simulink model "c221007_FCEV_CDCS"  (R2022b)
settings: Solver=ode4  StartTime=1  StopTime=size(Driving_cycle_v_kmph,1)  FixedStep=Auto  RelTol=1e-3  EnableMultiTasking=on
values from neighbouring files (symbols this model uses):
  Bat_eff_chg_average = 0.969    [FCEV_original_data.mat]
  Bat_eff_dis_average = 0.9632    [FCEV_original_data.mat]
  Bat_end_of_life_percent = 20    [FCEV_original_data.mat]
  Bat_I_chg_max = -120    [FCEV_original_data.mat]
  Bat_I_dis_max = 200    [FCEV_original_data.mat]
  Bat_nom_Ic = 2.5    [FCEV_original_data.mat]
  Bat_nom_SOC = 0.35    [FCEV_original_data.mat]
  Bat_nom_temp_oC = 25    [FCEV_original_data.mat]
  Bat_num_pa = 9    [FCEV_original_data.mat]
  Bat_num_se = 97    [FCEV_original_data.mat]
  Bat_ori_C1_chg_F = [397.526659684 455.660832136 435.08783522 460.845064365 457.605812374 417.289828504 416.373906992 359.741413056 321.561704819 1109.14132554 1165.67733205 1135.97600211 ... (72 elements, 9x8)]    [FCEV_original_data.mat]
  Bat_ori_C1_dis_F = [187.121968588 287.083505726 346.448009002 395.529439835 387.517274826 389.973134196 432.856765051 486.92921923 512.158935268 425.990733989 614.68708868 771.472592368 ... (72 elements, 9x8)]    [FCEV_original_data.mat]
  Bat_ori_C2_chg_F = [8748.48589695 7773.35875681 9404.86567646 8934.73981058 8290.58671366 7592.78422269 7759.44623103 7396.59043829 6151.35152293 16187.7227039 11721.8480541 13157.8579836 ... (72 elements, 9x8)]    [FCEV_original_data.mat]
  Bat_ori_C2_dis_F = [2939.81325553 4590.73311898 5504.93546413 5887.5077374 6534.37836712 7765.46899768 10584.7751706 10372.0508438 9238.72693885 5207.86390693 7911.43744944 8879.62137571 ... (72 elements, 9x8)]    [FCEV_original_data.mat]
  Bat_ori_cap_max_Ah = 20.7    [Config_c221218.m]    (also in Config_c230117.m; Config_c230321.m; FCEV_original_data.mat)
  Bat_ori_dUdt4 = [-0.303773584906 -0.249056603774 -0.115094339623 -0.0396226415094 0.0396226415094 0.0641509433962 0.107547169811 0.111320754717 0.0415094339623 0.0547169811321 0.130188679245]    [FCEV_original_data.mat]
  Bat_ori_R0_chg_O = [0.0771669453735 0.0731809311402 0.0726556782939 0.0729965156794 0.0731758310684 0.0742031005051 0.0721266921026 0.0714211058078 0.0714186176143 0.0374124505155 0.0354566732504 0.0345430657188 ... (72 elements, 9x8)]    [FCEV_original_data.mat]
  Bat_ori_R0_dis_O = [0.0819458671157 0.0812429476608 0.0803749674507 0.0805513601722 0.0838629023857 0.0850797840015 0.0829875518672 0.0826388888889 0.0812514106148 0.0428124986417 0.0424658903711 0.0428572670451 ... (72 elements, 9x8)]    [FCEV_original_data.mat]
  Bat_ori_R1_chg_O = [0.114339870884 0.105392753268 0.104421193553 0.109821896183 0.114868279838 0.123333154908 0.129174812826 0.149917249373 0.174896487845 0.0420560161846 0.0390948352938 0.0370122837364 ... (72 elements, 9x8)]    [FCEV_original_data.mat]
  Bat_ori_R1_dis_O = [0.304806399643 0.213604089624 0.171463520004 0.151183840498 0.140630862434 0.128795299077 0.116857791733 0.112567113582 0.106368362501 0.0943235089866 0.0730697254134 0.0611414736086 ... (72 elements, 9x8)]    [FCEV_original_data.mat]
  Bat_ori_R2_chg_O = [0.134518959939 0.17565045702 0.161100627268 0.189032232545 0.205639040497 0.226170473035 0.223651875822 0.181765694192 0.212966950836 0.073628872144 0.0788540822416 0.0792414571734 ... (72 elements, 9x8)]    [FCEV_original_data.mat]
  Bat_ori_R2_dis_O = [0.354968099904 0.285293035102 0.286338708953 0.298763853987 0.248762838155 0.178586175471 0.129047399775 0.188406991173 0.174494800676 0.131839238891 0.123225430215 0.132069033134 ... (72 elements, 9x8)]    [FCEV_original_data.mat]
  Bat_ori_SOC2 = [0 0.001 0.002 0.003 0.004 0.005 0.006 0.007 0.008 0.009 0.01 0.011 ... (1001 elements, 1x1001)]    [FCEV_original_data.mat]
  Bat_ori_SOC4 = [-0.00598301069999 0.0920117618231 0.190864167279 0.289083557951 0.387343788287 0.485011843502 0.5850485992 0.678163031937 0.774810095565 0.876684636119 0.972739524626]    [FCEV_original_data.mat]
  Bat_ori_Uoc_chg_V = [2.4478 2.54923264342 2.6007 2.6383 2.66953057366 2.69636321708 2.7197 2.74042850391 2.75906114733 2.77619379074 2.792 2.80675907757 ... (1001 elements, 1x1001)]    [FCEV_original_data.mat]
  Bat_ori_Uoc_dis_V = [1.9998 2.03916768329 2.24724374236 2.39700902919 2.48767431602 2.5476 2.5882 2.6202 2.64771773167 2.6719 2.6933 2.71251566192 ... (1001 elements, 1x1001)]    [FCEV_original_data.mat]
  Bat_ori_Uoc_V = [2.2238 2.29420016335 2.42397187118 2.5176545146 2.57860244484 2.62198160854 2.65395 2.68031425195 2.7033894395 2.72404689537 2.74265 2.75963736975 ... (1001 elements, 1x1001)]    [FCEV_original_data.mat]
  Bat_single_capacity_nom_Ah = 2.3    [FCEV_original_data.mat]
  Bat_SOC_cs_max = 0.4    [FCEV_original_data.mat]
  Bat_SOC_cs_min = 0.2    [FCEV_original_data.mat]
  Bat_SOC_ini = 0.3    [Config_c22100601.m]    (also in Config_c22100701.m; FCEV_original_data.mat = 0.45)
  Bat_SOC_max = 0.9    [FCEV_original_data.mat]
  Bat_SOC_min = 0.3    [FCEV_original_data.mat]
  Bat_temp_amb_oC = 25    [FCEV_original_data.mat]
  Bat_temp_cool_oC = 25    [FCEV_original_data.mat]
  Bat_U_avg_V = Bat_num_se*mean(Bat_ori_Uoc_V)    [Config_c22100601.m]    (also in Config_c22100701.m)
  DCAC_eff = 0.95    [FCEV_original_data.mat]
  DCDC_ori_eff = [0.95 0.96 0.97 0.976 0.98 0.978 0.973 0.962]    [FCEV_original_data.mat]
  DCDC_ori_power_kW = [0 10 20 30 40 50 60 70]    [FCEV_original_data.mat]
  FC_fuel_mass_ini_kg = 10    [FCEV_original_data.mat]
  FC_ori_eff = [0.1 0.33 0.492 0.533 0.559 0.596 0.591 0.562 0.508]    [FCEV_original_data.mat]
  FC_ori_fuel_rate_gps = [0 0.0505050505051 0.0846883468835 0.117260787992 0.149075730471 0.279642058166 0.423011844332 0.593119810202 0.820209973753]    [FCEV_original_data.mat]
  FC_ori_power_kW = [0 2 5 7.5 10 20 30 40 50]    [FCEV_original_data.mat]
  FC_power_max_kW = 50    [FCEV_original_data.mat]
  FC_power_min_kW = 0    [FCEV_original_data.mat]
  MC_eff_brk_average = 0.810578512397    [FCEV_original_data.mat]
  MC_eff_dri_average = 0.810578512397    [FCEV_original_data.mat]
  MC_inertia = 0.06    [FCEV_original_data.mat]
  MC_ori_eff = [0.7 0.78 0.85 0.86 0.81 0.82 0.79 0.78 0.78 0.78 0.78 0.7 ... (231 elements, 11x21)]    [FCEV_original_data.mat]
  MC_ori_power_brk_req_kW = [0 -28.3912930389 -56.7825860779 -85.1738791168 -113.565172156 -141.956465195 -170.347758234 -198.739051273 -227.130344311 -255.52163735 -283.912930389 0 ... (121 elements, 11x11)]    [FCEV_original_data.mat]
  MC_ori_power_dri_req_kW = [0 0 0 0 0 0 0 0 0 0 0 0 ... (121 elements, 11x11)]    [FCEV_original_data.mat]
  MC_ori_spd_rpm = [0 1000 2000 3000 4000 5000 6000 7000 8000 9000 10000]    [FCEV_original_data.mat]
  MC_ori_trq_brk_max_Nm = [-271.1368 -271.1368 -271.1368 -237.5159 -178.1369 -142.4824 -118.7579 -101.8119 -89.0685 -79.172 -71.1734]    [FCEV_original_data.mat]
  MC_ori_trq_brk_Nm = [-271.136848522 -244.02316367 -216.909478817 -189.795793965 -162.682109113 -135.568424261 -108.454739409 -81.3410545565 -54.2273697044 -27.1136848522 0]    [FCEV_original_data.mat]
  MC_ori_trq_dri_max_Nm = [271.1368 271.1368 271.1368 237.5159 178.1369 142.4824 118.7579 101.8119 89.0685 79.172 71.1734]    [FCEV_original_data.mat]
  MC_ori_trq_dri_Nm = [0 27.1136848522 54.2273697044 81.3410545565 108.454739409 135.568424261 162.682109113 189.795793965 216.909478817 244.02316367 271.136848522]    [FCEV_original_data.mat]
  MC_ori_trq_Nm = [-271.136848522 -244.02316367 -216.909478817 -189.795793965 -162.682109113 -135.568424261 -108.454739409 -81.3410545565 -54.2273697044 -27.1136848522 0 27.1136848522 ... (21 elements, 1x21)]    [FCEV_original_data.mat]
  MC_power_max_kW = 75    [FCEV_original_data.mat]
  MC_spd_max_rpm = 10000    [FCEV_original_data.mat]
  MC_spd_min_rpm = 0    [FCEV_original_data.mat]
  MC_spd_scale = 1    [FCEV_original_data.mat]
  MC_trq_scale = 1    [FCEV_original_data.mat]
  MC_U_min_V = 120    [FCEV_original_data.mat]
  Road_u = 0.75    [FCEV_original_data.mat]
  S_r = floor(max(Sr_SOC_process(:,1))):-1:0    [Config_c22100601.m]    (also in Config_c22100701.m)
  Time_sample = 60    [Driving_cycle_recognition_data.mat]
  Trip_distance_total_km = sum(Driving_cycle_v_kmph(:,2)/3.6)/1000    [Config_c22100601.m]    (also in Config_c22100701.m)
  usd2rmb = 7.116    [Config_c22100601.m]    (also in Config_c22100701.m; Config_c221106.m = 6; Config_c221112.m = 6; Config_c221127.m = 6)
  Veh_air_density_kgpm2 = 1.2    [FCEV_original_data.mat]
  Veh_brk_front = [1 0.6 0.608 0.61 0.618 0.624 0.636 0.645 0.655]    [FCEV_original_data.mat]
  Veh_brk_z = [0.1 0.2 0.3 0.4 0.5 0.6 0.7 0.8 0.9]    [FCEV_original_data.mat]
  Veh_brk_z_max = 0.7    [FCEV_original_data.mat]
  Veh_brk_z_min = 0.1    [FCEV_original_data.mat]
  Veh_coeff_drag = 0.312    [FCEV_original_data.mat]
  Veh_coeff_roll = 0.00863    [FCEV_original_data.mat]
  Veh_final_drive_inertia = 0.1105    [FCEV_original_data.mat]
  Veh_final_drive_ratio = 3.47    [FCEV_original_data.mat]
  Veh_frontal_area_m2 = 2.06    [FCEV_original_data.mat]
  Veh_gravity_acc_ms2 = 9.81    [FCEV_original_data.mat]
  Veh_mass_cargo_kg = 113    [FCEV_original_data.mat]
  Veh_mass_curb_kg = 1157    [FCEV_original_data.mat]
  Veh_mech_eff = 0.9    [FCEV_original_data.mat]
  Veh_rotary_mass_conversion_factor = 1.05    [FCEV_original_data.mat]
  Veh_size_cg_height_m = 0.53    [FCEV_original_data.mat]
  Veh_wheel_inertia = 3.1039    [FCEV_original_data.mat]
  Veh_wheel_radius_m = 0.313    [FCEV_original_data.mat]
  Veh_wt_frac_front = 0.5    [FCEV_original_data.mat]
undefined symbols (not defined in the file or in its folder): alpha, Bat_ori_temp, Sr_e
libraries: neural x10
(part 4 of 5)

== system c221007_FCEV_CDCS/电池模型/Electrical Model/Max power in W (Battery pack level)/Max power in W (Battery pack level)1 ==
  SOC : Inport
  1-D Lookup Table : Lookup_n-D  NumberOfTableDimensions=1  BreakpointsForDimension1=Bat_ori_SOC2  Table=Bat_ori_Uoc_V  RndMeth=Simplest
  1-D Lookup Table1 : Lookup_n-D  NumberOfTableDimensions=1  BreakpointsForDimension1=Bat_ori_SOC2  Table=Bat_ori_Uoc_V  RndMeth=Simplest
  Constant : Constant  Value=MC_U_min_V
  Constant1 : Constant  Value=0.001
  Constant2 : Constant  Value=0
  Constant3 : Constant  Value=Bat_SOC_min
  Constant4 : Constant  Value=Bat_SOC_max
  Gain : Gain  Gain=0.5  SaturateOnIntegerOverflow=on  OutDataTypeStr=Inherit: Same as input  ParamDataTypeStr=Inherit: Same as input
  MinMax1 : MinMax  Function=max  Inputs=3  InputSameDT=on  SaturateOnIntegerOverflow=on
  Mux : Mux  Inputs=3
  Mux3 : Mux  Inputs=3
  Mux5 : Mux  Inputs=3
  Product3 : Product  InputSameDT=on  RndMeth=Zero  SaturateOnIntegerOverflow=on  OutDataTypeStr=Inherit: Same as first input
  R0,cell->R0,bat : Gain  Gain=Bat_num_se/Bat_num_pa  SaturateOnIntegerOverflow=on  OutDataTypeStr=Inherit: Same as input  ParamDataTypeStr=Inherit: Same as input
  R0,cell->R0,bat1 : Gain  Gain=Bat_num_se/Bat_num_pa  SaturateOnIntegerOverflow=on  OutDataTypeStr=Inherit: Same as input  ParamDataTypeStr=Inherit: Same as input
  Relational Operator : RelationalOperator  Operator=>
  Switch : Switch  Threshold=eps
  Uoc,cell->Uoc,bat : Gain  Gain=Bat_num_se  SaturateOnIntegerOverflow=on  OutDataTypeStr=Inherit: Same as input  ParamDataTypeStr=Inherit: Same as input
  Uoc,cell->Uoc,bat1 : Gain  Gain=Bat_num_se  SaturateOnIntegerOverflow=on  OutDataTypeStr=Inherit: Same as input  ParamDataTypeStr=Inherit: Same as input
  Voc-I*R : Fcn  Expr=u[2]-u[1]*u[3]
  iabs min=(Voc-Vmax)/R : Fcn  Expr=(u(1)-u(2))/u(3)
  max power corresponding to minimum voltage : Fcn  Expr=(u[1]-u[2])*u[2]/u[3]
  max ess discharge pwr : Outport  InitialOutput=0
  max ess charge pwr : Outport  Port=2  InitialOutput=0
  wires:
  Voc-I*R/1 -> Product3/2
  iabs min=(Voc-Vmax)/R/1 -> Product3/1, Mux3/1
  Mux3/1 -> Voc-I*R/1
  Mux5/1 -> iabs min=(Voc-Vmax)/R/1
  Uoc,cell->Uoc,bat1/1 -> Mux5/2
  Switch/1 -> max ess discharge pwr/1
  SOC/1 -> Relational Operator/1
  Constant2/1 -> Switch/3
  max power corresponding to minimum voltage/1 -> Switch/1
  [Bat_Uoc_V] -> Mux3/2, Mux5/1, Gain/1, Mux/1
  MinMax1/1 -> Mux/2
  Gain/1 -> MinMax1/1
  Mux/1 -> max power corresponding to minimum voltage/1
  Constant/1 -> MinMax1/2
  Constant1/1 -> Relational Operator/2
  Uoc,cell->Uoc,bat/1 -> MinMax1/3
  Relational Operator/1 -> Switch/2
  [Bat_R0_dis_O] -> R0,cell->R0,bat/1
  R0,cell->R0,bat/1 -> Mux/3
  [Bat_R0_chg_O] -> R0,cell->R0,bat1/1
  R0,cell->R0,bat1/1 -> Mux5/3, Mux3/3
  Constant3/1 -> 1-D Lookup Table/1
  1-D Lookup Table/1 -> Uoc,cell->Uoc,bat/1
  Constant4/1 -> 1-D Lookup Table1/1
  1-D Lookup Table1/1 -> Uoc,cell->Uoc,bat1/1
  Product3/1 -> max ess charge pwr/1

== system c221007_FCEV_CDCS/电池模型/Electrical Model/Parameter Lookup2/Lookup C1 ==
  SOC : Inport
  T : Inport  Port=2
  P : Inport  Port=3
  Lookup Table (2-D) C1_c : Lookup2D  RowIndex=Bat_ori_SOC_chg  ColumnIndex=Bat_ori_temp_oC  Table=Bat_ori_C1_chg_F  SaturateOnIntegerOverflow=off  InputSameDT=off
  Lookup Table (2-D) C1_d : Lookup2D  RowIndex=Bat_ori_SOC_dis  ColumnIndex=Bat_ori_temp_oC  Table=Bat_ori_C1_dis_F  SaturateOnIntegerOverflow=off  InputSameDT=off
  Switch : Switch  SaturateOnIntegerOverflow=off  InputSameDT=off
  C1 : Outport
  wires:
  T/1 -> Lookup Table (2-D) C1_c/2, Lookup Table (2-D) C1_d/2
  SOC/1 -> Lookup Table (2-D) C1_c/1, Lookup Table (2-D) C1_d/1
  Lookup Table (2-D) C1_c/1 -> Switch/3
  Lookup Table (2-D) C1_d/1 -> Switch/1
  Switch/1 -> C1/1
  P/1 -> Switch/2

== system c221007_FCEV_CDCS/电池模型/Electrical Model/Parameter Lookup2/Lookup C2 ==
  SOC : Inport
  T : Inport  Port=2
  P : Inport  Port=3
  Lookup Table (2-D) C2_c : Lookup2D  RowIndex=Bat_ori_SOC_chg  ColumnIndex=Bat_ori_temp_oC  Table=Bat_ori_C2_chg_F  SaturateOnIntegerOverflow=off  InputSameDT=off
  Lookup Table (2-D) C2_d : Lookup2D  RowIndex=Bat_ori_SOC_dis  ColumnIndex=Bat_ori_temp_oC  Table=Bat_ori_C2_dis_F  SaturateOnIntegerOverflow=off  InputSameDT=off
  Switch : Switch  SaturateOnIntegerOverflow=off  InputSameDT=off
  C2 : Outport
  wires:
  T/1 -> Lookup Table (2-D) C2_c/2, Lookup Table (2-D) C2_d/2
  SOC/1 -> Lookup Table (2-D) C2_c/1, Lookup Table (2-D) C2_d/1
  Lookup Table (2-D) C2_c/1 -> Switch/3
  Lookup Table (2-D) C2_d/1 -> Switch/1
  Switch/1 -> C2/1
  P/1 -> Switch/2

== system c221007_FCEV_CDCS/电池模型/Electrical Model/Parameter Lookup2/Lookup R1 ==
  SOC : Inport
  T : Inport  Port=2
  P : Inport  Port=3
  Lookup Table (2-D) R1_c : Lookup2D  RowIndex=Bat_ori_SOC_chg  ColumnIndex=Bat_ori_temp_oC  Table=Bat_ori_R1_chg_O  SaturateOnIntegerOverflow=off  InputSameDT=off
  Lookup Table (2-D) R1_d : Lookup2D  RowIndex=Bat_ori_SOC_dis  ColumnIndex=Bat_ori_temp_oC  Table=Bat_ori_R1_dis_O  SaturateOnIntegerOverflow=off  InputSameDT=off
  Switch : Switch  SaturateOnIntegerOverflow=off  InputSameDT=off
  R1 : Outport
  wires:
  T/1 -> Lookup Table (2-D) R1_d/2, Lookup Table (2-D) R1_c/2
  SOC/1 -> Lookup Table (2-D) R1_d/1, Lookup Table (2-D) R1_c/1
  Lookup Table (2-D) R1_c/1 -> Switch/3
  Lookup Table (2-D) R1_d/1 -> Switch/1
  P/1 -> Switch/2
  Switch/1 -> R1/1

== system c221007_FCEV_CDCS/电池模型/Electrical Model/Parameter Lookup2/Lookup R2 ==
  SOC1 : Inport
  T : Inport  Port=2
  P : Inport  Port=3
  Lookup Table (2-D) R2_c : Lookup2D  RowIndex=Bat_ori_SOC_chg  ColumnIndex=Bat_ori_temp_oC  Table=Bat_ori_R2_chg_O  SaturateOnIntegerOverflow=off  InputSameDT=off
  Lookup Table (2-D) R2_d : Lookup2D  RowIndex=Bat_ori_SOC_dis  ColumnIndex=Bat_ori_temp_oC  Table=Bat_ori_R2_dis_O  SaturateOnIntegerOverflow=off  InputSameDT=off
  Switch : Switch  SaturateOnIntegerOverflow=off  InputSameDT=off
  R2 : Outport
  wires:
  T/1 -> Lookup Table (2-D) R2_d/2, Lookup Table (2-D) R2_c/2
  SOC1/1 -> Lookup Table (2-D) R2_d/1, Lookup Table (2-D) R2_c/1
  Lookup Table (2-D) R2_c/1 -> Switch/3
  Lookup Table (2-D) R2_d/1 -> Switch/1
  P/1 -> Switch/2
  Switch/1 -> R2/1

== system c221007_FCEV_CDCS/电池模型/Electrical Model/Parameter Lookup2/Lookup Rs ==
  SOC : Inport
  T : Inport  Port=2
  Lookup Table (2-D) R0_c : Lookup2D  RowIndex=Bat_ori_SOC_chg  ColumnIndex=Bat_ori_temp_oC  Table=Bat_ori_R0_chg_O  SaturateOnIntegerOverflow=off  InputSameDT=off
  Lookup Table (2-D) R0_d : Lookup2D  RowIndex=Bat_ori_SOC_dis  ColumnIndex=Bat_ori_temp_oC  Table=Bat_ori_R0_dis_O  SaturateOnIntegerOverflow=off  InputSameDT=off
  Mux : Mux  Inputs=2
  R0 : Outport
  tag scope: Bat_R0_chg_O=global, Bat_R0_dis_O=global
  wires:
  Lookup Table (2-D) R0_d/1 -> Mux/1, [Bat_R0_dis_O]
  Lookup Table (2-D) R0_c/1 -> Mux/2, [Bat_R0_chg_O]
  SOC/1 -> Lookup Table (2-D) R0_c/1, Lookup Table (2-D) R0_d/1
  T/1 -> Lookup Table (2-D) R0_c/2, Lookup Table (2-D) R0_d/2
  Mux/1 -> R0/1

== system c221007_FCEV_CDCS/电池模型/Electrical Model/Parameter Lookup2/Lookup Uoc ==
  SOC : Inport
  P : Inport  Port=2
  Switch : Switch  SaturateOnIntegerOverflow=off  InputSameDT=off
  VOC-chg : Lookup_n-D  NumberOfTableDimensions=1  BreakpointsForDimension1=Bat_ori_SOC2  BreakpointsForDimension2=Bat_ori_temp  Table=Bat_ori_Uoc_chg_V  InternalRulePriority=Speed  RndMeth=Simplest
  VOC-dischg : Lookup_n-D  NumberOfTableDimensions=1  BreakpointsForDimension1=Bat_ori_SOC2  BreakpointsForDimension2=Bat_ori_temp  Table=Bat_ori_Uoc_dis_V  InternalRulePriority=Speed  RndMeth=Simplest
  Uoc : Outport
  wires:
  SOC/1 -> VOC-chg/1, VOC-dischg/1
  VOC-chg/1 -> Switch/3
  VOC-dischg/1 -> Switch/1
  Switch/1 -> Uoc/1
  P/1 -> Switch/2

== system c221007_FCEV_CDCS/电池模型/Electrical Model/SOC Calculation/CD//CS mode judgement ==
  note: 当前SOC
  SOC : Inport
  Constant2 : Constant  Value=Bat_SOC_min
  Logical Operator1 : Logic  Operator=NOT  AllPortsSameDT=off  OutDataTypeStr=boolean
  Relational Operator : RelationalOperator  OutDataTypeStr=boolean  InputSameDT=off
  Scope1 : Scope
  To Workspace2 : ToWorkspace  VariableName=Bat_charge_sustaining_on  SampleTime=-1
  tag scope: Bat_charge_sustaining_on=global
  wires:
  SOC/1 -> Relational Operator/1
  Constant2/1 -> Relational Operator/2
  Logical Operator1/1 -> Scope1/1, To Workspace2/1, [Bat_charge_sustaining_on]
  Relational Operator/1 -> Logical Operator1/1

== system c221007_FCEV_CDCS/电池模型/Subsystem/Capacity Degradation Model (Cell)1/计算实际寿命 ==
  note: 参考文献：A control-oriented cycle-life model for hybrid electric vehicle lithiumion batteries
  note: Beta
  note: Alpha
  温度 : Inport
  倍率 : Inport  Port=2
  SOC : Inport  Port=3
  -31700+163.3*Ic : Sum  InputSameDT=on  SaturateOnIntegerOverflow=on  OutDataTypeStr=Inherit: Same as first input
  Alpha*SOC+Beta1 : Sum  InputSameDT=on  SaturateOnIntegerOverflow=on  OutDataTypeStr=Inherit: Same as first input
  Alpha3 : Constant  Value=2896.6
  Alpha4 : Constant  Value=2649.5
  Beta3 : Constant  Value=7411.2
  Beta4 : Constant  Value=6022.2
  Constant : Constant  Value=-31500
  Constant1 : Constant  Value=152.5
  Constant2 : Constant  Value=273.15
  Fcn2 : Fcn  Expr=u^(1/0.57)
  Math Function : Math  Operator=reciprocal  SignedPower=on
  Math Function1 : Math  Operator=reciprocal  SignedPower=on
  Math Function2 : Math  SignedPower=on
  R : Constant  Value=8.314
  R*T : Product  InputSameDT=on  RndMeth=Zero  SaturateOnIntegerOverflow=on  OutDataTypeStr=Inherit: Same as first input
  Switch3 : Switch  Criteria=u2 > Threshold  Threshold=0.45
  Switch4 : Switch  Criteria=u2 > Threshold  Threshold=0.45
  severity factor function : Product  InputSameDT=on  RndMeth=Zero  SaturateOnIntegerOverflow=on  OutDataTypeStr=Inherit: Same as first input
  x : Product  InputSameDT=on  RndMeth=Zero  SaturateOnIntegerOverflow=on  OutDataTypeStr=Inherit: Same as first input
  x1 : Product  InputSameDT=on  RndMeth=Zero  SaturateOnIntegerOverflow=on  OutDataTypeStr=Inherit: Same as first input
  x2 : Product  InputSameDT=on  RndMeth=Zero  SaturateOnIntegerOverflow=on  OutDataTypeStr=Inherit: Same as first input
  ×1 : Product  InputSameDT=on  RndMeth=Zero  SaturateOnIntegerOverflow=on  OutDataTypeStr=Inherit: Same as first input
  ℃->开氏温度(绝对温度) : Sum  InputSameDT=on  SaturateOnIntegerOverflow=on  OutDataTypeStr=Inherit: Same as first input
  电池标准状态寿命 : ToWorkspace  VariableName=Bat_life_nom  SampleTime=-1
  电池终止寿命(%) : Constant  Value=Bat_end_of_life_percent
  Bat_life_nom : Outport
  wires:
  R/1 -> R*T/1
  ℃->开氏温度(绝对温度)/1 -> R*T/2
  Constant/1 -> -31700+163.3*Ic/1
  x/1 -> -31700+163.3*Ic/2
  Constant1/1 -> x/1
  -31700+163.3*Ic/1 -> x1/1
  R*T/1 -> Math Function/1
  Math Function/1 -> x1/2
  x1/1 -> Math Function2/1
  温度/1 -> ℃->开氏温度(绝对温度)/1
  Constant2/1 -> ℃->开氏温度(绝对温度)/2
  倍率/1 -> x/2
  Math Function2/1 -> severity factor function/1
  Alpha*SOC+Beta1/1 -> severity factor function/2
  severity factor function/1 -> Math Function1/1
  电池终止寿命(%)/1 -> x2/1
  Math Function1/1 -> x2/2
  x2/1 -> Fcn2/1
  Fcn2/1 -> Bat_life_nom/1, 电池标准状态寿命/1
  SOC/1 -> Switch4/2, ×1/1, Switch3/2
  Alpha4/1 -> Switch3/1
  Alpha3/1 -> Switch3/3
  Beta4/1 -> Switch4/1
  Beta3/1 -> Switch4/3
  Switch3/1 -> ×1/2
  Switch4/1 -> Alpha*SOC+Beta1/2
  ×1/1 -> Alpha*SOC+Beta1/1

== system c221007_FCEV_CDCS/电池模型/Subsystem/Capacity Degradation Model (Cell)1/计算电池寿命(标准条件下) ==
  note: 参考文献：A control-oriented cycle-life model for hybrid electric vehicle lithiumion batteries
  note: Beta
  note: Alpha
  标准温度 : Inport
  标准倍率 : Inport  Port=2
  标准SOC : Inport  Port=3
  -31500+152.5*Ic : Sum  InputSameDT=on  SaturateOnIntegerOverflow=on  OutDataTypeStr=Inherit: Same as first input
  Alpha*SOC+Beta : Sum  InputSameDT=on  SaturateOnIntegerOverflow=on  OutDataTypeStr=Inherit: Same as first input
  Alpha3 : Constant  Value=2896.6
  Alpha4 : Constant  Value=2649.5
  Beta3 : Constant  Value=7411.2
  Beta4 : Constant  Value=6022.2
  Constant : Constant  Value=-31500
  Constant1 : Constant  Value=152.5
  Constant2 : Constant  Value=273.15
  Fcn2 : Fcn  Expr=u^(1/0.57)
  Math Function : Math  Operator=reciprocal  SignedPower=on
  Math Function1 : Math  Operator=reciprocal  SignedPower=on
  Math Function2 : Math  SignedPower=on
  R : Constant  Value=8.314
  R*T : Product  InputSameDT=on  RndMeth=Zero  SaturateOnIntegerOverflow=on  OutDataTypeStr=Inherit: Same as first input
  Switch3 : Switch  Criteria=u2 > Threshold  Threshold=0.45
  Switch4 : Switch  Criteria=u2 > Threshold  Threshold=0.45
  severity factor function : Product  InputSameDT=on  RndMeth=Zero  SaturateOnIntegerOverflow=on  OutDataTypeStr=Inherit: Same as first input
  x : Product  InputSameDT=on  RndMeth=Zero  SaturateOnIntegerOverflow=on  OutDataTypeStr=Inherit: Same as first input
  x1 : Product  InputSameDT=on  RndMeth=Zero  SaturateOnIntegerOverflow=on  OutDataTypeStr=Inherit: Same as first input
  x2 : Product  InputSameDT=on  RndMeth=Zero  SaturateOnIntegerOverflow=on  OutDataTypeStr=Inherit: Same as first input
  ×1 : Product  InputSameDT=on  RndMeth=Zero  SaturateOnIntegerOverflow=on  OutDataTypeStr=Inherit: Same as first input
  ℃->开氏温度(绝对温度) : Sum  InputSameDT=on  SaturateOnIntegerOverflow=on  OutDataTypeStr=Inherit: Same as first input
  电池实际状态寿命 : ToWorkspace  VariableName=Bat_life_act  SampleTime=-1
  电池终止寿命(%) : Constant  Value=Bat_end_of_life_percent
  Bat_life_act : Outport
  wires:
  R/1 -> R*T/1
  ℃->开氏温度(绝对温度)/1 -> R*T/2
  Constant/1 -> -31500+152.5*Ic/1
  x/1 -> -31500+152.5*Ic/2
  Constant1/1 -> x/1
  -31500+152.5*Ic/1 -> x1/1
  R*T/1 -> Math Function/1
  Math Function/1 -> x1/2
  x1/1 -> Math Function2/1
  标准温度/1 -> ℃->开氏温度(绝对温度)/1
  Constant2/1 -> ℃->开氏温度(绝对温度)/2
  标准倍率/1 -> x/2
  Math Function2/1 -> severity factor function/1
  Alpha*SOC+Beta/1 -> severity factor function/2
  severity factor function/1 -> Math Function1/1
  电池终止寿命(%)/1 -> x2/1
  Math Function1/1 -> x2/2
  x2/1 -> Fcn2/1
  Fcn2/1 -> Bat_life_act/1, 电池实际状态寿命/1
  标准SOC/1 -> Switch4/2, ×1/1, Switch3/2
  Alpha4/1 -> Switch3/1
  Alpha3/1 -> Switch3/3
  Beta4/1 -> Switch4/1
  Beta3/1 -> Switch4/3
  Switch3/1 -> ×1/2
  Switch4/1 -> Alpha*SOC+Beta/2
  ×1/1 -> Alpha*SOC+Beta/1

== system c221007_FCEV_CDCS/电池模型/Subsystem/Electrical Model1/Current calculation ==
  note: #:电池单体水平
  note: R0chg
  note: R0dis
  Voc : Inport
  Rint : Inport  Port=2
  limited output power (W) : Inport  Port=3
  Constant : Constant  Value=Bat_I_chg_max
  Constant1 : Constant  Value=Bat_I_dis_max
  Constant2 : Constant  Value=0
  Demux : Demux  Outputs=2
  Ibty=(Voc-(Voc^2-4RPbty)^.5) ----------------------------- (2*R) : Fcn  Expr=(u[2]-(u[2]^2-4*u[1]*u[3])^.5)/(2*u[3])
  Ibty=(Voc-(Voc^2-4RPbty)^.5) ----------------------------- (2*R)1 : Fcn  Expr=(u[2]-(u[2]^2-4*u[1]*u[3])^.5)/(2*u[3])
  MinMax : MinMax  Inputs=2
  MinMax1 : MinMax  Function=max  Inputs=2
  Mux : Mux  Inputs=2
  Mux1 : Mux  Inputs=3
  Mux2 : Mux  Inputs=3
  Pbat->Pcell : Gain  Gain=1/(Bat_num_pa*Bat_num_se)  SaturateOnIntegerOverflow=on  OutDataTypeStr=Inherit: Same as input  ParamDataTypeStr=Inherit: Same as input
  Scope : Scope
  Scope1 : Scope
  Switch : Switch  Criteria=u2 > Threshold
  Switch1 : Switch  Criteria=u2 > Threshold  SaturateOnIntegerOverflow=off  InputSameDT=off
  Switch2 : Switch  Criteria=u2 > Threshold
  I_dis (A) I_chg (A) Cell : Outport  InitialOutput=0
  I (A) Cell : Outport  Port=2  InitialOutput=0
  wires:
  Rint/1 -> Demux/1
  limited output power (W)/1 -> Pbat->Pcell/1
  Pbat->Pcell/1 -> Switch/1, Switch/2, Switch2/3, Switch2/2, Switch1/2
  Mux1/1 -> Ibty=(Voc-(Voc^2-4RPbty)^.5) ----------------------------- (2*R)/1
  Demux/1 -> Mux1/3
  Voc/1 -> Mux1/2, Mux2/2
  Demux/2 -> Mux2/3
  Mux2/1 -> Ibty=(Voc-(Voc^2-4RPbty)^.5) ----------------------------- (2*R)1/1
  Ibty=(Voc-(Voc^2-4RPbty)^.5) ----------------------------- (2*R)/1 -> MinMax/2
  Constant1/1 -> MinMax/1
  Ibty=(Voc-(Voc^2-4RPbty)^.5) ----------------------------- (2*R)1/1 -> MinMax1/1
  Constant/1 -> MinMax1/2
  MinMax/1 -> Switch1/1, Mux/1
  MinMax1/1 -> Mux/2, Switch1/3
  Mux/1 -> Scope/1, I_dis (A) I_chg (A) Cell/1
  Switch1/1 -> Scope1/1, I (A) Cell/1
  Switch/1 -> Mux1/1
  Switch2/1 -> Mux2/1
  Constant2/1 -> Switch/3, Switch2/1

== system c221007_FCEV_CDCS/电池模型/Subsystem/Electrical Model1/Entropic Heat ==
  note: 用于计算可逆热
  T : Inport
  SOC : Inport  Port=2
  Constant : Constant  Value=273
  Ent heat : Product  RndMeth=Zero
  Scope : Scope
  Sum2 : Sum  Inputs=|++
  dudT : Lookup  InputValues=Bat_ori_SOC4  Table=Bat_ori_dUdt4  SaturateOnIntegerOverflow=off
  mV->V : Gain  Gain=1/1000
  HG_ent : Outport
  wires:
  Sum2/1 -> Ent heat/2
  Constant/1 -> Sum2/2
  T/1 -> Sum2/1
  dudT/1 -> Ent heat/1
  Ent heat/1 -> mV->V/1
  SOC/1 -> dudT/1
  mV->V/1 -> Scope/1, HG_ent/1

== system c221007_FCEV_CDCS/电池模型/Subsystem/Electrical Model1/Limited power (Battery pack level) ==
  SOC : Inport
  Pbty : Inport  Port=2
  " " : RelationalOperator  Operator=>  OutDataTypeStr=boolean  InputSameDT=off
  " 1" : RelationalOperator  Operator=<  OutDataTypeStr=boolean  InputSameDT=off
  " 3" : Constant  Value=0.95
  Add : Sum
  Constant : Constant  Value=eps
  Constant1 : Constant  Value=eps
  Constant{2..5} (4 alike) : Constant  Value=0
  Logical Operator : Logic  Operator=OR  AllPortsSameDT=off  OutDataTypeStr=boolean
  Logical Operator1 : Logic  AllPortsSameDT=off  OutDataTypeStr=boolean
  Memory1 : Memory  InitialCondition=Bat_SOC_ini  InheritSampleTime=on
  Relational Operator : RelationalOperator  Operator=>  OutDataTypeStr=boolean  InputSameDT=off
  Relational Operator1 : RelationalOperator  OutDataTypeStr=boolean  InputSameDT=off
  Scope : Scope
  Scope1 : Scope  NumInputPorts=2
  Scope2 : Scope  NumInputPorts=2
  Scope3 : Scope
  Switch{,1..3} (4 alike) : Switch  Criteria=u2 > Threshold  Threshold=eps  SaturateOnIntegerOverflow=off  InputSameDT=off
  "Pbty, limited W" : Outport  InitialOutput=0
  wires:
  Memory1/1 -> Relational Operator/1, Relational Operator1/1, Scope3/1
  Constant/1 -> Relational Operator/2
  Relational Operator/1 -> Logical Operator/1
  Switch3/1 -> Scope2/2, " 1"/1, Switch1/3
  Constant1/1 -> " "/2
  " "/1 -> Logical Operator/2
  Logical Operator/1 -> Switch/2
  Constant2/1 -> Switch/3
  " 3"/1 -> Relational Operator1/2
  Relational Operator1/1 -> Logical Operator1/1
  Logical Operator1/1 -> Switch1/2
  Constant3/1 -> Switch1/1
  Constant4/1 -> " 1"/2
  " 1"/1 -> Logical Operator1/2
  Switch2/1 -> Scope2/1, " "/1, Switch/1
  Add/1 -> Scope/1, "Pbty, limited W"/1
  Switch/1 -> Scope1/1, Add/1
  Switch1/1 -> Add/2, Scope1/2
  Pbty/1 -> Switch3/3, Switch3/2, Switch2/1, Switch2/2
  Constant5/1 -> Switch3/1, Switch2/3
  SOC/1 -> Memory1/1

== system c221007_FCEV_CDCS/电池模型/Subsystem/Electrical Model1/Max power in W (Battery pack level) ==
  Constant3 : Constant  Value=Bat_I_dis_max
  Constant4 : Constant  Value=Bat_I_chg_max
  Max power in W (Battery pack level)1 : Subsystem
  Mux1 : Mux  Inputs=3
  Mux2 : Mux  Inputs=3
  Product : Product  InputSameDT=on  RndMeth=Zero  SaturateOnIntegerOverflow=on  OutDataTypeStr=Inherit: Same as first input
  Product1 : Product  InputSameDT=on  RndMeth=Zero  SaturateOnIntegerOverflow=on  OutDataTypeStr=Inherit: Same as first input
  R0,cell->R0,bat : Gain  Gain=Bat_num_se/Bat_num_pa  SaturateOnIntegerOverflow=on  OutDataTypeStr=Inherit: Same as input  ParamDataTypeStr=Inherit: Same as input
  R0,cell->R0,bat1 : Gain  Gain=Bat_num_se/Bat_num_pa  SaturateOnIntegerOverflow=on  OutDataTypeStr=Inherit: Same as input  ParamDataTypeStr=Inherit: Same as input
  fun : Fcn  Expr=u[2]-u[1]*u[3]
  fun1 : Fcn  Expr=u[2]-u[1]*u[3]
  max ess discharge pwr : Outport  InitialOutput=0
  max ess charge pwr : Outport  Port=2  InitialOutput=0
  wires:
  [Bat_R0_dis_O] -> R0,cell->R0,bat/1
  [Bat_R0_chg_O] -> R0,cell->R0,bat1/1
  Constant4/1 -> Product1/1, Mux2/1
  Constant3/1 -> Product/1, Mux1/1
  R0,cell->R0,bat/1 -> Mux1/3
  [Bat_Uoc_V] -> Mux2/2, Mux1/2
  Mux1/1 -> fun/1
  R0,cell->R0,bat1/1 -> Mux2/3
  Mux2/1 -> fun1/1
  fun/1 -> Product/2
  Product/1 -> max ess discharge pwr/1
  fun1/1 -> Product1/2
  Product1/1 -> max ess charge pwr/1

== system c221007_FCEV_CDCS/电池模型/Subsystem/Electrical Model1/Parameter Lookup2 ==
  note: #Cell层面
  SOC : Inport
  T : Inport  Port=2
  P : Inport  Port=3
  Gain{1..5} (5 alike) : Gain
  Lookup C1 : Subsystem
  Lookup C2 : Subsystem
  Lookup R1 : Subsystem
  Lookup R2 : Subsystem
  Lookup Rs : Subsystem
  Lookup Uoc : Subsystem
  Uoc : Outport
  R1 : Outport  Port=2
  C1 : Outport  Port=3
  R2 : Outport  Port=4
  C2 : Outport  Port=5
  R0 : Outport  Port=6
  wires:
  SOC/1 -> Lookup Rs/1(SOC), Lookup R1/1(SOC), Lookup C1/1(SOC), Lookup Uoc/1(SOC), Lookup C2/1(SOC), Lookup R2/1(SOC1)
  T/1 -> Lookup Rs/2(T), Lookup R1/2(T), Lookup C1/2(T), Lookup C2/2(T), Lookup R2/2(T)
  P/1 -> Lookup R1/3(P), Lookup C1/3(P), Lookup C2/3(P), Lookup Uoc/2(P), Lookup R2/3(P)
  Gain3/1 -> C1/1
  Lookup C2/1(C2) -> Gain4/1
  Gain4/1 -> C2/1
  Gain2/1 -> R2/1
  Lookup R2/1(R2) -> Gain2/1
  Gain1/1 -> R1/1
  Lookup R1/1(R1) -> Gain1/1
  Lookup C1/1(C1) -> Gain3/1
  Lookup Uoc/1(Uoc) -> Gain5/1
  Gain5/1 -> Uoc/1
  Lookup Rs/1(R0) -> R0/1

== system c221007_FCEV_CDCS/电池模型/Subsystem/Electrical Model1/SOC Calculation ==
  note: 充电
  note: 放电
  note: #:电池组水平
  I_dis (A) I_chg (A) : Inport
  (sec->hrs) : Gain  Gain=1/3600  SaturateOnIntegerOverflow=on  OutDataTypeStr=Inherit: Same as input  ParamDataTypeStr=Inherit: Same as input
  0 <= SOC <= 1 : Saturate  UpperLimit=1  LowerLimit=eps
  Add5 : Sum  Inputs=-+
  Add6 : Sum  Inputs=-+
  Bat SOC0 : Constant  Value=Bat_SOC_ini
  Bat chg eff : Constant  Value=Bat_eff_chg_average
  Bat dis eff : Constant  Value=Bat_eff_dis_average
  CD/CS mode judgement : Subsystem
  Demux : Demux  Outputs=2
  Divide1 : Product  Inputs=*/
  Divide3 : Product  Inputs=**
  Divide4 : Product  Inputs=*/
  Icell->Ibat : Gain  Gain=Bat_num_pa  SaturateOnIntegerOverflow=on  OutDataTypeStr=Inherit: Same as input  ParamDataTypeStr=Inherit: Same as input
  Icell->Ibat1 : Gain  Gain=Bat_num_pa  SaturateOnIntegerOverflow=on  OutDataTypeStr=Inherit: Same as input  ParamDataTypeStr=Inherit: Same as input
  Integrator1 : Integrator  InitialCondition=eps
  Integrator6 : Integrator
  Integrator7 : Integrator
  Product3 : Product  RndMeth=Zero
  Product4 : Product  RndMeth=Zero
  Q0 : Constant  Value=Bat_ori_cap_max_Ah
  Scope : Scope
  Switch : Switch  Criteria=u2 > Threshold  SaturateOnIntegerOverflow=off  InputSameDT=off
  To Workspace3 : ToWorkspace  VariableName=Energy_bat_consume_kWh  SaveFormat=Timeseries  SampleTime=-1
  Ws->kWh : Gain  Gain=-1/(1000*3600)
  Ws->kWh1 : Gain  Gain=-1/(1000*3600)
  SOC : Outport  InitialOutput=0
  wires:
  0 <= SOC <= 1/1 -> CD/CS mode judgement/1(SOC), SOC/1
  I_dis (A) I_chg (A)/1 -> Scope/1, Demux/1
  Demux/1 -> Icell->Ibat/1
  Demux/2 -> Icell->Ibat1/1
  Divide3/1 -> Switch/2, Product3/1, Switch/1
  Icell->Ibat/1 -> Divide3/1
  Bat dis eff/1 -> Divide3/2
  Bat chg eff/1 -> Divide4/2
  Icell->Ibat1/1 -> Divide4/1
  Divide4/1 -> Product4/2, Switch/3
  Add5/1 -> 0 <= SOC <= 1/1
  [Bat_Uoc_V] -> Product4/1, Product3/2
  Add6/1 -> To Workspace3/1
  Product3/1 -> Integrator6/1
  Integrator6/1 -> Ws->kWh/1
  Ws->kWh/1 -> Add6/1
  Product4/1 -> Integrator7/1
  Integrator7/1 -> Ws->kWh1/1
  Ws->kWh1/1 -> Add6/2
  Switch/1 -> (sec->hrs)/1
  (sec->hrs)/1 -> Integrator1/1
  Integrator1/1 -> Divide1/1
  Q0/1 -> Divide1/2
  Bat SOC0/1 -> Add5/2
  Divide1/1 -> Add5/1

== system c221007_FCEV_CDCS/电池模型/Subsystem/Electrical Model1/U0 ==
  R0 : Inport
  I : Inport  Port=2
  Demux : Demux  Outputs=2
  Switch : Switch  Criteria=u2 > Threshold  SaturateOnIntegerOverflow=off  InputSameDT=off
  U0=I*R0 : Product  RndMeth=Zero
  U0 : Outport
  wires:
  I/1 -> U0=I*R0/2, Switch/2
  R0/1 -> Demux/1
  Demux/1 -> Switch/1
  Demux/2 -> Switch/3
  Switch/1 -> U0=I*R0/1
  U0=I*R0/1 -> U0/1

== system c221007_FCEV_CDCS/电池模型/Subsystem/Electrical Model1/U1&U1 ==
  note: -V2/(C2*R2)+I/C2
  note: -V1/(C1*R1)+I/C1
  R1 : Inport
  C1 : Inport  Port=2
  R2 : Inport  Port=3
  C2 : Inport  Port=4
  I : Inport  Port=5
  Ib/C1 : Product  Inputs=*/  RndMeth=Zero
  Ib/C2 : Product  Inputs=*/  RndMeth=Zero
  Memory : Memory  InitialCondition=eps  InheritSampleTime=on
  Memory1 : Memory  InitialCondition=eps  InheritSampleTime=on
  R1*C1 : Product  Inputs=**  RndMeth=Zero
  R2*C2 : Product  Inputs=**  RndMeth=Zero
  Scope : Scope  NumInputPorts=2
  Scope1 : Scope
  Sum1 : Sum
  Sum2 : Sum  Inputs=|-+
  Sum3 : Sum  Inputs=+-|
  Sum4 : Sum
  U1/(R1*C1) : Product  Inputs=*/  RndMeth=Zero
  U2/(R2*C2) : Product  Inputs=*/  RndMeth=Zero
  U1 : Outport
  U2 : Outport  Port=2
  wires:
  C1/1 -> R1*C1/1, Ib/C1/2
  I/1 -> Scope1/1, Ib/C2/1, Ib/C1/1
  R1/1 -> R1*C1/2
  R1*C1/1 -> U1/(R1*C1)/2
  U1/(R1*C1)/1 -> Sum3/2
  Ib/C1/1 -> Sum3/1
  R2/1 -> R2*C2/1
  C2/1 -> Ib/C2/2, R2*C2/2
  R2*C2/1 -> U2/(R2*C2)/2
  Ib/C2/1 -> Sum2/2
  U2/(R2*C2)/1 -> Sum2/1
  Memory/1 -> U1/(R1*C1)/1, Sum1/2
  Memory1/1 -> Sum4/1, U2/(R2*C2)/1
  Sum3/1 -> Sum1/1
  Sum1/1 -> Scope/1, Memory/1, U1/1
  Sum2/1 -> Sum4/2
  Sum4/1 -> Scope/2, Memory1/1, U2/1

== system c221007_FCEV_CDCS/电池模型/Subsystem/Thermal Model1/Calculation ==
  Cc1 : Constant  Value=62.7
  Cs : Constant  Value=4.5
  "Rc " : Constant  Value=1.94
  Rc*Cc : Product  Inputs=**  RndMeth=Zero
  Rc*Cs : Product  Inputs=**  RndMeth=Zero
  Rs : Constant  Value=3.19
  Rs*Cs : Product  Inputs=**  RndMeth=Zero
  Cc : Outport
  RcCc : Outport  Port=2
  RsCs : Outport  Port=3
  RcCs : Outport  Port=4
  wires:
  Cc1/1 -> Cc/1, Rc*Cc/1
  "Rc "/1 -> Rc*Cc/2, Rc*Cs/1
  Rc*Cc/1 -> RcCc/1
  Cs/1 -> Rs*Cs/1, Rc*Cs/2
  Rs/1 -> Rs*Cs/2
  Rc*Cs/1 -> RcCs/1
  Rs*Cs/1 -> RsCs/1

== system c221007_FCEV_CDCS/能量管理策略 (ECMS+SQP)/FC on/no-lag Reset Integrator/dt ==
  Clock : Clock
  Memory1 : Memory  InitialCondition=-1
  Sum1 : Sum  Inputs=+-  InputSameDT=on  SaturateOnIntegerOverflow=on  OutDataTypeStr=Inherit: Same as first input
  out_1 : Outport  InitialOutput=0
  wires:
  Clock/1 -> Sum1/1, Memory1/1
  Memory1/1 -> Sum1/2
  Sum1/1 -> out_1/1

== system c221007_FCEV_CDCS/行驶工况相关/Custom Neural Network/Layer 1/Delays 1 ==
  "p{1}" : Inport  PortDimensions=3
      mask Display: e = 0.06;c1 = [120 230 180]/255;c2 = ([120 230 180]+0)/(256+128);c3 = ([120 230 180]+128)/(256+128);patch([0 1 1 0],[0 0 1 1],c1);patch([0 1 1 1-e 1-e 0+e],[0 0 1 1-e 0+e 0+e],c2);patch([0 0 1 1-e 0+e 0+e],[0 1 1 1-e 1-e 0+e],c3);plot([0 1 1 0 0],[0 0 1 1 0]);
  mux : Mux  Inputs=1
      mask Display: e = 0.06;c1 = [120 150 230]/255;c2 = ([120 150 230]+0)/383;c3 = ([120 150 230]+128)/383;patch([0 1 1 0],[0 0 1 1],c1);patch([0 1 1 1-e 1-e 0+e],[0 0 1 1-e 0+e 0+e],c2);patch([0 0 1 1-e 0+e 0+e],[0 1 1 1-e 1-e 0+e],c3);plot([0 1 1 0 0],[0 0 1 1 0]);disp('Mux')
  "pd{1,1}" : Outport
      mask Display: e = 0.06;c1 = [120 230 180]/255;c2 = ([120 230 180]+0)/(256+128);c3 = ([120 230 180]+128)/(256+128);patch([0 1 1 0],[0 0 1 1],c1);patch([0 1 1 1-e 1-e 0+e],[0 0 1 1-e 0+e 0+e],c2);patch([0 0 1 1-e 0+e 0+e],[0 1 1 1-e 1-e 0+e],c3);plot([0 1 1 0 0],[0 0 1 1 0]);
  wires:
  "p{1}"/1 -> mux/1
  mux/1 -> "pd{1,1}"/1

== system c221007_FCEV_CDCS/行驶工况相关/Custom Neural Network/Layer 1/IW{1,1} ==
  "pd{1,1}" : Inport  PortDimensions=3
      mask Display: e = 0.06;c1 = [120 230 180]/255;c2 = ([120 230 180]+0)/(256+128);c3 = ([120 230 180]+128)/(256+128);patch([0 1 1 0],[0 0 1 1],c1);patch([0 1 1 1-e 1-e 0+e],[0 0 1 1-e 0+e 0+e],c2);patch([0 0 1 1-e 0+e 0+e],[0 1 1 1-e 1-e 0+e],c3);plot([0 1 1 0 0],[0 0 1 1 0]);
  "IW{1,1}(1,:)'" : Constant  Value=[-22.664682786208438;32.76807488580922;-18.369833338195413]
      mask Display: e = 0.06;c1 = [120 150 230]/255;c2 = ([120 150 230]+0)/383;c3 = ([120 150 230]+128)/383;patch([0 1 1 0],[0 0 1 1],c1);patch([0 1 1 1-e 1-e 0+e],[0 0 1 1-e 0+e 0+e],c2);patch([0 0 1 1-e 0+e 0+e],[0 1 1 1-e 1-e 0+e],c3);plot([0 1 1 0 0],[0 0 1 1 0]);disp('Weights');
  "IW{1,1}(2,:)'" : Constant  Value=[-21.468554017248199;52.490015103408602;-22.886328621274419]
      mask Display: e = 0.06;c1 = [120 150 230]/255;c2 = ([120 150 230]+0)/383;c3 = ([120 150 230]+128)/383;patch([0 1 1 0],[0 0 1 1],c1);patch([0 1 1 1-e 1-e 0+e],[0 0 1 1-e 0+e 0+e],c2);patch([0 0 1 1-e 0+e 0+e],[0 1 1 1-e 1-e 0+e],c3);plot([0 1 1 0 0],[0 0 1 1 0]);disp('Weights');
  "IW{1,1}(3,:)'" : Constant  Value=[-36.237551671476247;66.088181838731572;-31.430403718789275]
      mask Display: e = 0.06;c1 = [120 150 230]/255;c2 = ([120 150 230]+0)/383;c3 = ([120 150 230]+128)/383;patch([0 1 1 0],[0 0 1 1],c1);patch([0 1 1 1-e 1-e 0+e],[0 0 1 1-e 0+e 0+e],c2);patch([0 0 1 1-e 0+e 0+e],[0 1 1 1-e 1-e 0+e],c3);plot([0 1 1 0 0],[0 0 1 1 0]);disp('Weights');
  "IW{1,1}(4,:)'" : Constant  Value=[-27.763414762552355;53.30625106546244;-25.296683174595962]
      mask Display: e = 0.06;c1 = [120 150 230]/255;c2 = ([120 150 230]+0)/383;c3 = ([120 150 230]+128)/383;patch([0 1 1 0],[0 0 1 1],c1);patch([0 1 1 1-e 1-e 0+e],[0 0 1 1-e 0+e 0+e],c2);patch([0 0 1 1-e 0+e 0+e],[0 1 1 1-e 1-e 0+e],c3);plot([0 1 1 0 0],[0 0 1 1 0]);disp('Weights');
  "IW{1,1}(5,:)'" : Constant  Value=[-27.762870447003099;53.298594948653026;-25.384972141376959]
      mask Display: e = 0.06;c1 = [120 150 230]/255;c2 = ([120 150 230]+0)/383;c3 = ([120 150 230]+128)/383;patch([0 1 1 0],[0 0 1 1],c1);patch([0 1 1 1-e 1-e 0+e],[0 0 1 1-e 0+e 0+e],c2);patch([0 0 1 1-e 0+e 0+e],[0 1 1 1-e 1-e 0+e],c3);plot([0 1 1 0 0],[0 0 1 1 0]);disp('Weights');
  Mux : Mux  Inputs=5
      mask Display: e = 0.06;c1 = [120 150 230]/255;c2 = ([120 150 230]+0)/383;c3 = ([120 150 230]+128)/383;patch([0 1 1 0],[0 0 1 1],c1);patch([0 1 1 1-e 1-e 0+e],[0 0 1 1-e 0+e 0+e],c2);patch([0 0 1 1-e 0+e 0+e],[0 1 1 1-e 1-e 0+e],c3);plot([0 1 1 0 0],[0 0 1 1 0]);disp('Mux');
  negdist{1..5} (5 alike) : neural/Weight Functions/negdist
  "iz{1,1}" : Outport
      mask Display: e = 0.06;c1 = [120 230 180]/255;c2 = ([120 230 180]+0)/(256+128);c3 = ([120 230 180]+128)/(256+128);patch([0 1 1 0],[0 0 1 1],c1);patch([0 1 1 1-e 1-e 0+e],[0 0 1 1-e 0+e 0+e],c2);patch([0 0 1 1-e 0+e 0+e],[0 1 1 1-e 1-e 0+e],c3);plot([0 1 1 0 0],[0 0 1 1 0]);
  wires:
  "IW{1,1}(1,:)'"/1 -> negdist1/1
  "pd{1,1}"/1 -> negdist1/2, negdist2/2, negdist3/2, negdist4/2, negdist5/2
  negdist1/1 -> Mux/1
  "IW{1,1}(2,:)'"/1 -> negdist2/1
  negdist2/1 -> Mux/2
  "IW{1,1}(3,:)'"/1 -> negdist3/1
  negdist3/1 -> Mux/3
  "IW{1,1}(4,:)'"/1 -> negdist4/1
  negdist4/1 -> Mux/4
  "IW{1,1}(5,:)'"/1 -> negdist5/1
  negdist5/1 -> Mux/5
  Mux/1 -> "iz{1,1}"/1

== system c221007_FCEV_CDCS/行驶工况相关/Custom Neural Network/Layer 2/Delays 1 ==
  "p{2}" : Inport  PortDimensions=5
      mask Display: e = 0.06;c1 = [120 230 180]/255;c2 = ([120 230 180]+0)/(256+128);c3 = ([120 230 180]+128)/(256+128);patch([0 1 1 0],[0 0 1 1],c1);patch([0 1 1 1-e 1-e 0+e],[0 0 1 1-e 0+e 0+e],c2);patch([0 0 1 1-e 0+e 0+e],[0 1 1 1-e 1-e 0+e],c3);plot([0 1 1 0 0],[0 0 1 1 0]);
  mux : Mux  Inputs=1
      mask Display: e = 0.06;c1 = [120 150 230]/255;c2 = ([120 150 230]+0)/383;c3 = ([120 150 230]+128)/383;patch([0 1 1 0],[0 0 1 1],c1);patch([0 1 1 1-e 1-e 0+e],[0 0 1 1-e 0+e 0+e],c2);patch([0 0 1 1-e 0+e 0+e],[0 1 1 1-e 1-e 0+e],c3);plot([0 1 1 0 0],[0 0 1 1 0]);disp('Mux')
  "pd{2,1}" : Outport
      mask Display: e = 0.06;c1 = [120 230 180]/255;c2 = ([120 230 180]+0)/(256+128);c3 = ([120 230 180]+128)/(256+128);patch([0 1 1 0],[0 0 1 1],c1);patch([0 1 1 1-e 1-e 0+e],[0 0 1 1-e 0+e 0+e],c2);patch([0 0 1 1-e 0+e 0+e],[0 1 1 1-e 1-e 0+e],c3);plot([0 1 1 0 0],[0 0 1 1 0]);
  wires:
  "p{2}"/1 -> mux/1
  mux/1 -> "pd{2,1}"/1

== system c221007_FCEV_CDCS/行驶工况相关/Custom Neural Network/Layer 2/LW{2,1} ==
  "ad{2,1}" : Inport  PortDimensions=5
      mask Display: e = 0.06;c1 = [120 230 180]/255;c2 = ([120 230 180]+0)/(256+128);c3 = ([120 230 180]+128)/(256+128);patch([0 1 1 0],[0 0 1 1],c1);patch([0 1 1 1-e 1-e 0+e],[0 0 1 1-e 0+e 0+e],c2);patch([0 0 1 1-e 0+e 0+e],[0 1 1 1-e 1-e 0+e],c3);plot([0 1 1 0 0],[0 0 1 1 0]);
  "IW{2,1}(1,:)'" : Constant  Value=[1;0;0;0;0]
      mask Display: e = 0.06;c1 = [120 150 230]/255;c2 = ([120 150 230]+0)/383;c3 = ([120 150 230]+128)/383;patch([0 1 1 0],[0 0 1 1],c1);patch([0 1 1 1-e 1-e 0+e],[0 0 1 1-e 0+e 0+e],c2);patch([0 0 1 1-e 0+e 0+e],[0 1 1 1-e 1-e 0+e],c3);plot([0 1 1 0 0],[0 0 1 1 0]);disp('weights');
  "IW{2,1}(2,:)'" : Constant  Value=[0;1;0;0;0]
      mask Display: e = 0.06;c1 = [120 150 230]/255;c2 = ([120 150 230]+0)/383;c3 = ([120 150 230]+128)/383;patch([0 1 1 0],[0 0 1 1],c1);patch([0 1 1 1-e 1-e 0+e],[0 0 1 1-e 0+e 0+e],c2);patch([0 0 1 1-e 0+e 0+e],[0 1 1 1-e 1-e 0+e],c3);plot([0 1 1 0 0],[0 0 1 1 0]);disp('weights');
  "IW{2,1}(3,:)'" : Constant  Value=[0;0;1;1;1]
      mask Display: e = 0.06;c1 = [120 150 230]/255;c2 = ([120 150 230]+0)/383;c3 = ([120 150 230]+128)/383;patch([0 1 1 0],[0 0 1 1],c1);patch([0 1 1 1-e 1-e 0+e],[0 0 1 1-e 0+e 0+e],c2);patch([0 0 1 1-e 0+e 0+e],[0 1 1 1-e 1-e 0+e],c3);plot([0 1 1 0 0],[0 0 1 1 0]);disp('weights');
  Mux : Mux  Inputs=3
      mask Display: e = 0.06;c1 = [120 150 230]/255;c2 = ([120 150 230]+0)/383;c3 = ([120 150 230]+128)/383;patch([0 1 1 0],[0 0 1 1],c1);patch([0 1 1 1-e 1-e 0+e],[0 0 1 1-e 0+e 0+e],c2);patch([0 0 1 1-e 0+e 0+e],[0 1 1 1-e 1-e 0+e],c3);plot([0 1 1 0 0],[0 0 1 1 0]);disp('Mux');
  dotprod1 : neural/Weight Functions/dotprod
  dotprod2 : neural/Weight Functions/dotprod
  dotprod3 : neural/Weight Functions/dotprod
  "lz{2,1}" : Outport
      mask Display: e = 0.06;c1 = [120 230 180]/255;c2 = ([120 230 180]+0)/(256+128);c3 = ([120 230 180]+128)/(256+128);patch([0 1 1 0],[0 0 1 1],c1);patch([0 1 1 1-e 1-e 0+e],[0 0 1 1-e 0+e 0+e],c2);patch([0 0 1 1-e 0+e 0+e],[0 1 1 1-e 1-e 0+e],c3);plot([0 1 1 0 0],[0 0 1 1 0]);
  wires:
  "IW{2,1}(1,:)'"/1 -> dotprod1/1
  "ad{2,1}"/1 -> dotprod1/2, dotprod2/2, dotprod3/2
  dotprod1/1 -> Mux/1
  "IW{2,1}(2,:)'"/1 -> dotprod2/1
  dotprod2/1 -> Mux/2
  "IW{2,1}(3,:)'"/1 -> dotprod3/1
  dotprod3/1 -> Mux/3
  Mux/1 -> "lz{2,1}"/1

== system c221007_FCEV_CDCS/电池模型/Subsystem/Electrical Model1/Max power in W (Battery pack level)/Max power in W (Battery pack level)1 ==
  SOC : Inport
  1-D Lookup Table : Lookup_n-D  NumberOfTableDimensions=1  BreakpointsForDimension1=Bat_ori_SOC2  Table=Bat_ori_Uoc_V  RndMeth=Simplest
  1-D Lookup Table1 : Lookup_n-D  NumberOfTableDimensions=1  BreakpointsForDimension1=Bat_ori_SOC2  Table=Bat_ori_Uoc_V  RndMeth=Simplest
  Constant : Constant  Value=MC_U_min_V
  Constant1 : Constant  Value=0.001
  Constant2 : Constant  Value=0
  Constant3 : Constant  Value=Bat_SOC_min
  Constant4 : Constant  Value=Bat_SOC_max
  Gain : Gain  Gain=0.5  SaturateOnIntegerOverflow=on  OutDataTypeStr=Inherit: Same as input  ParamDataTypeStr=Inherit: Same as input
  MinMax1 : MinMax  Function=max  Inputs=3  InputSameDT=on  SaturateOnIntegerOverflow=on
  Mux : Mux  Inputs=3
  Mux3 : Mux  Inputs=3
  Mux5 : Mux  Inputs=3
  Product3 : Product  InputSameDT=on  RndMeth=Zero  SaturateOnIntegerOverflow=on  OutDataTypeStr=Inherit: Same as first input
  R0,cell->R0,bat : Gain  Gain=Bat_num_se/Bat_num_pa  SaturateOnIntegerOverflow=on  OutDataTypeStr=Inherit: Same as input  ParamDataTypeStr=Inherit: Same as input
  R0,cell->R0,bat1 : Gain  Gain=Bat_num_se/Bat_num_pa  SaturateOnIntegerOverflow=on  OutDataTypeStr=Inherit: Same as input  ParamDataTypeStr=Inherit: Same as input
  Relational Operator : RelationalOperator  Operator=>
  Switch : Switch  Threshold=eps
  Uoc,cell->Uoc,bat : Gain  Gain=Bat_num_se  SaturateOnIntegerOverflow=on  OutDataTypeStr=Inherit: Same as input  ParamDataTypeStr=Inherit: Same as input
  Uoc,cell->Uoc,bat1 : Gain  Gain=Bat_num_se  SaturateOnIntegerOverflow=on  OutDataTypeStr=Inherit: Same as input  ParamDataTypeStr=Inherit: Same as input
  Voc-I*R : Fcn  Expr=u[2]-u[1]*u[3]
  iabs min=(Voc-Vmax)/R : Fcn  Expr=(u(1)-u(2))/u(3)
  max power corresponding to minimum voltage : Fcn  Expr=(u[1]-u[2])*u[2]/u[3]
  max ess discharge pwr : Outport  InitialOutput=0
  max ess charge pwr : Outport  Port=2  InitialOutput=0
  wires:
  Voc-I*R/1 -> Product3/2
  iabs min=(Voc-Vmax)/R/1 -> Product3/1, Mux3/1
  Mux3/1 -> Voc-I*R/1
  Mux5/1 -> iabs min=(Voc-Vmax)/R/1
  Uoc,cell->Uoc,bat1/1 -> Mux5/2
  Switch/1 -> max ess discharge pwr/1
  SOC/1 -> Relational Operator/1
  Constant2/1 -> Switch/3
  max power corresponding to minimum voltage/1 -> Switch/1
  [Bat_Uoc_V] -> Mux3/2, Mux5/1, Gain/1, Mux/1
  MinMax1/1 -> Mux/2
  Gain/1 -> MinMax1/1
  Mux/1 -> max power corresponding to minimum voltage/1
  Constant/1 -> MinMax1/2
  Constant1/1 -> Relational Operator/2
  Uoc,cell->Uoc,bat/1 -> MinMax1/3
  Relational Operator/1 -> Switch/2
  [Bat_R0_dis_O] -> R0,cell->R0,bat/1
  R0,cell->R0,bat/1 -> Mux/3
  [Bat_R0_chg_O] -> R0,cell->R0,bat1/1
  R0,cell->R0,bat1/1 -> Mux5/3, Mux3/3
  Constant3/1 -> 1-D Lookup Table/1
  1-D Lookup Table/1 -> Uoc,cell->Uoc,bat/1
  Constant4/1 -> 1-D Lookup Table1/1
  1-D Lookup Table1/1 -> Uoc,cell->Uoc,bat1/1
  Product3/1 -> max ess charge pwr/1

== system c221007_FCEV_CDCS/电池模型/Subsystem/Electrical Model1/Parameter Lookup2/Lookup C1 ==
  SOC : Inport
  T : Inport  Port=2
  P : Inport  Port=3
  Lookup Table (2-D) C1_c : Lookup2D  RowIndex=Bat_ori_SOC_chg  ColumnIndex=Bat_ori_temp_oC  Table=Bat_ori_C1_chg_F  SaturateOnIntegerOverflow=off  InputSameDT=off
  Lookup Table (2-D) C1_d : Lookup2D  RowIndex=Bat_ori_SOC_dis  ColumnIndex=Bat_ori_temp_oC  Table=Bat_ori_C1_dis_F  SaturateOnIntegerOverflow=off  InputSameDT=off
  Switch : Switch  SaturateOnIntegerOverflow=off  InputSameDT=off
  C1 : Outport
  wires:
  T/1 -> Lookup Table (2-D) C1_c/2, Lookup Table (2-D) C1_d/2
  SOC/1 -> Lookup Table (2-D) C1_c/1, Lookup Table (2-D) C1_d/1
  Lookup Table (2-D) C1_c/1 -> Switch/3
  Lookup Table (2-D) C1_d/1 -> Switch/1
  Switch/1 -> C1/1
  P/1 -> Switch/2

== system c221007_FCEV_CDCS/电池模型/Subsystem/Electrical Model1/Parameter Lookup2/Lookup C2 ==
  SOC : Inport
  T : Inport  Port=2
  P : Inport  Port=3
  Lookup Table (2-D) C2_c : Lookup2D  RowIndex=Bat_ori_SOC_chg  ColumnIndex=Bat_ori_temp_oC  Table=Bat_ori_C2_chg_F  SaturateOnIntegerOverflow=off  InputSameDT=off
  Lookup Table (2-D) C2_d : Lookup2D  RowIndex=Bat_ori_SOC_dis  ColumnIndex=Bat_ori_temp_oC  Table=Bat_ori_C2_dis_F  SaturateOnIntegerOverflow=off  InputSameDT=off
  Switch : Switch  SaturateOnIntegerOverflow=off  InputSameDT=off
  C2 : Outport
  wires:
  T/1 -> Lookup Table (2-D) C2_c/2, Lookup Table (2-D) C2_d/2
  SOC/1 -> Lookup Table (2-D) C2_c/1, Lookup Table (2-D) C2_d/1
  Lookup Table (2-D) C2_c/1 -> Switch/3
  Lookup Table (2-D) C2_d/1 -> Switch/1
  Switch/1 -> C2/1
  P/1 -> Switch/2

== system c221007_FCEV_CDCS/电池模型/Subsystem/Electrical Model1/Parameter Lookup2/Lookup R1 ==
  SOC : Inport
  T : Inport  Port=2
  P : Inport  Port=3
  Lookup Table (2-D) R1_c : Lookup2D  RowIndex=Bat_ori_SOC_chg  ColumnIndex=Bat_ori_temp_oC  Table=Bat_ori_R1_chg_O  SaturateOnIntegerOverflow=off  InputSameDT=off
  Lookup Table (2-D) R1_d : Lookup2D  RowIndex=Bat_ori_SOC_dis  ColumnIndex=Bat_ori_temp_oC  Table=Bat_ori_R1_dis_O  SaturateOnIntegerOverflow=off  InputSameDT=off
  Switch : Switch  SaturateOnIntegerOverflow=off  InputSameDT=off
  R1 : Outport
  wires:
  T/1 -> Lookup Table (2-D) R1_d/2, Lookup Table (2-D) R1_c/2
  SOC/1 -> Lookup Table (2-D) R1_d/1, Lookup Table (2-D) R1_c/1
  Lookup Table (2-D) R1_c/1 -> Switch/3
  Lookup Table (2-D) R1_d/1 -> Switch/1
  P/1 -> Switch/2
  Switch/1 -> R1/1

== system c221007_FCEV_CDCS/电池模型/Subsystem/Electrical Model1/Parameter Lookup2/Lookup R2 ==
  SOC1 : Inport
  T : Inport  Port=2
  P : Inport  Port=3
  Lookup Table (2-D) R2_c : Lookup2D  RowIndex=Bat_ori_SOC_chg  ColumnIndex=Bat_ori_temp_oC  Table=Bat_ori_R2_chg_O  SaturateOnIntegerOverflow=off  InputSameDT=off
  Lookup Table (2-D) R2_d : Lookup2D  RowIndex=Bat_ori_SOC_dis  ColumnIndex=Bat_ori_temp_oC  Table=Bat_ori_R2_dis_O  SaturateOnIntegerOverflow=off  InputSameDT=off
  Switch : Switch  SaturateOnIntegerOverflow=off  InputSameDT=off
  R2 : Outport
  wires:
  T/1 -> Lookup Table (2-D) R2_d/2, Lookup Table (2-D) R2_c/2
  SOC1/1 -> Lookup Table (2-D) R2_d/1, Lookup Table (2-D) R2_c/1
  Lookup Table (2-D) R2_c/1 -> Switch/3
  Lookup Table (2-D) R2_d/1 -> Switch/1
  P/1 -> Switch/2
  Switch/1 -> R2/1
